simulink model "spring_damping_mass_System_2dof"  (R2017a)
settings: Solver=ode45  StartTime=0.0  StopTime=20  RelTol=1e-3  EnableMultiTasking=on
undefined symbols (not defined in the file): c1, c2, k1, k2, m1, m2
settings Model: Creator=edward  LastModifiedBy=edward
settings DataIOCC: LimitDataPoints=on  SaveFormat=Array
settings OptimizationCC: LifeSpan=inf
settings DebuggingCC: UnderspecifiedInitializationDetection=Classic  MergeDetectMultiDrivingBlocksExec=none  SolverPrmCheckMsg=warning  SFUnexpectedBacktrackingDiag=warning  SFNoUnconditionalDefaultTransitionDiag=warning  SFExecutionAtInitializationDiag=none
settings HardwareCC: ProdBitPerPointer=32  ProdBitPerSizeT=32  ProdBitPerPtrDiffT=32  ProdLargestAtomicFloat=None  ProdIntDivRoundTo=Undefined  ProdEndianess=Unspecified  ProdWordSize=32  ProdHWDeviceType=32-bit Generic
settings ModelReferenceCC: PropagateSignalLabelsOutOfModel=off
settings GRTTargetCC: TargetLangStandard=C89/C90 (ANSI)  GeneratePreprocessorConditionals=Disable all
settings ConfigComp: CovMetricSettings=dw  CovHtmlReporting=on  CovSaveCumulativeToWorkspaceVar=on  CovSaveSingleToWorkspaceVar=on  CovExternalEMLEnable=off

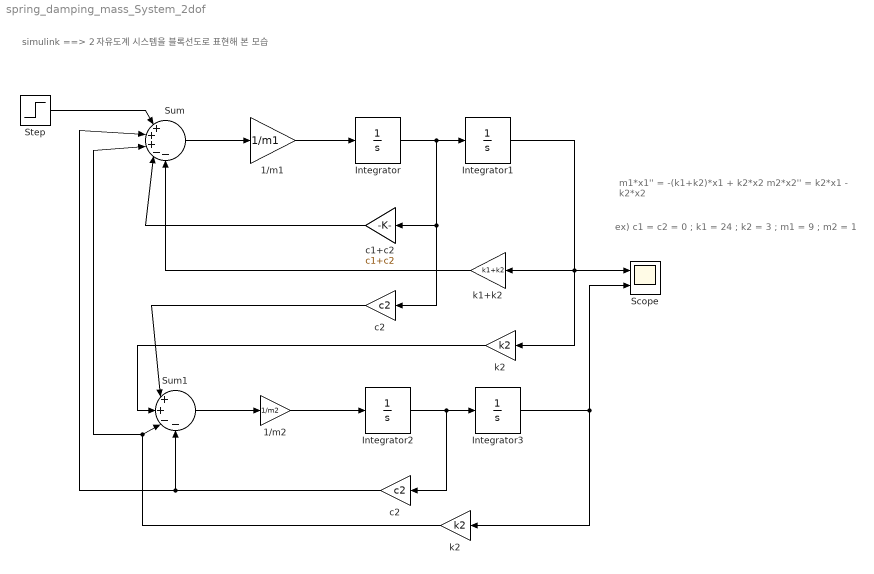
== system spring_damping_mass_System_2dof ==
  note: m1*x1'' =  -(k1+k2)*x1 + k2*x2
      | m2*x2'' =    k2*x1     - k2*x2
  note: simulink ==> 2 자유도계 시스템을 블록선도로 표현해 본 모습
  note: ex) c1 = c2 = 0 ; k1 = 24 ; k2 = 3 ; m1 = 9 ; m2 = 1
  1/m1 : Gain  Gain=1/m1
  1/m2 : Gain  Gain=1/m2
  Integrator : Integrator
  Integrator1 : Integrator  InitialCondition=1
  Integrator2 : Integrator
  Integrator3 : Integrator
  Scope : Scope  NumInputPorts=2
  Step : Step  Time=0  SampleTime=0
  Sum : Sum  Inputs=|+++--
  Sum1 : Sum  Inputs=|++--
  c1+c2 : Gain  Gain=c1+c2
  c2 : Gain  Gain=c2
  "c2 " : Gain  Gain=c2
  k1+k2 : Gain  Gain=k1+k2
  k2 : Gain  Gain=k2
  "k2 " : Gain  Gain=k2
  wires:
  Integrator/1 -> c1+c2/1, "c2 "/1, Integrator1/1
  Integrator1/1 -> k1+k2/1, "k2 "/1, Scope/1
  1/m1/1 -> Integrator/1
  Sum/1 -> 1/m1/1
  k1+k2/1 -> Sum/5
  Integrator2/1 -> c2/1, Integrator3/1
  Integrator3/1 -> k2/1, Scope/2
  1/m2/1 -> Integrator2/1
  Sum1/1 -> 1/m2/1
  c2/1 -> Sum1/4, Sum/2
  k2/1 -> Sum/3, Sum1/3
  "c2 "/1 -> Sum1/1
  "k2 "/1 -> Sum1/2
  Step/1 -> Sum/1
  c1+c2/1 -> Sum/4
